simulink model "B2B_spv"  (R2017a)
settings: Solver=VariableStepAuto  StartTime=0.0  StopTime=.2  MaxStep=1e-4  RelTol=1e-3
libraries: powerlib x77, powerlib_meascontrol x11, dsparch4 x2
(part 1 of 2)
settings Model: Creator=erich  LastModifiedBy=erich

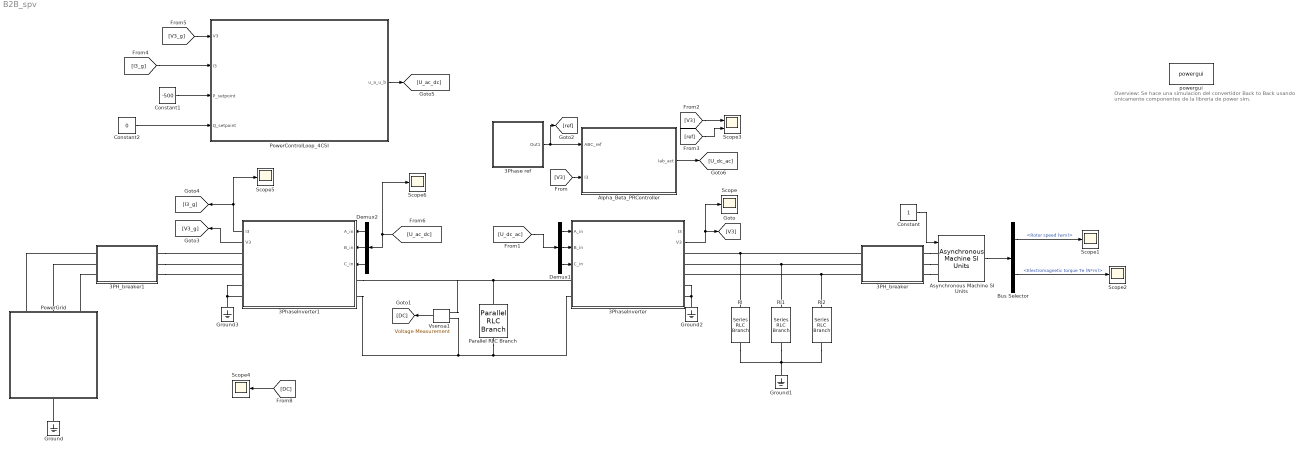
== system B2B_spv ==
  note: Overview:
      | Se hace una simulacion del convertidor
      | Back to Back usando unicamente componentes de la
      | libreria de power sim.
  3PH_breaker : Subsystem  mask{start_time=.3}
      mask prompts: start_time "Time Before  Conection"
      mask Display:
      | port_label('lconn', 1, 'a')
      | port_label('lconn', 2, 'b')
      | port_label('lconn', 3, 'c')
      | port_label('rconn', 1, 'A')
      | port_label('rconn', 2, 'B')
      | port_label('rconn', 3, 'C')
      | 
      | text(.3, .3, '3 \Phi Breaker', 'texmode', 'on')
      | 
      | plot([.3 .43], [.55 .55])
      | plot([.57 .7], [.55 .55])
      | 
      | x = -.09:.01:.09;
      | y = sqrt(.1.^2 - x.^2)*1.7;
      | 
      | plot(x+.5, .55+y)
  3PH_breaker1 : Subsystem  mask{start_time=2e-3}
      mask prompts: start_time "Time Before  Conection"
      mask Display:
      | port_label('lconn', 1, 'a')
      | port_label('lconn', 2, 'b')
      | port_label('lconn', 3, 'c')
      | port_label('rconn', 1, 'A')
      | port_label('rconn', 2, 'B')
      | port_label('rconn', 3, 'C')
      | 
      | text(.3, .3, '3 \Phi Breaker', 'texmode', 'on')
      | 
      | plot([.3 .43], [.55 .55])
      | plot([.57 .7], [.55 .55])
      | 
      | x = -.09:.01:.09;
      | y = sqrt(.1.^2 - x.^2)*1.7;
      | 
      | plot(x+.5, .55+y)
  3Phase ref : Subsystem  mask{f=60, A=170}
      mask prompts: f "Frequency (Hz)"; A "Amplitude"
      mask Display:
      | port_label('output', 1, 'sine(t)_{abc}', 'texmode', 'on')
      | 
      | 
      | plot([0:.001:.3], sin([0:.001:.3]*2*pi*10)/10+.8)
      | plot([0:.001:.3], sin([0:.001:.3]*2*pi*10)/10+.5)
      | plot([0:.001:.3], sin([0:.001:.3]*2*pi*10)/10+.2)
  3PhaseInverter : Subsystem  mask(Power SIM Block){f_sw=10000, start_Delay=.3, filter=[2e-3 .01 4.7e-6 .01]}
      mask prompts: f_sw "Switching Frequency (Hz)"; start_Delay "Converter starting delay"; filter "Parametros filtros [Lf, rLf, Cf, rCf]"
      mask help: Este es un convertidor trifasico implementado a la partir de la topologia 3 leg converter. Se emplea un filtro LC trifasico para suavizar la salida del inversor. puede hacer operacion bidireccional (DC -> AC y AC -> DC).
      mask DialogControl DescTextVar Prompt: Configuracion Del Inversor Trifasico. Switching Frequency corresponde a la frecuencia de conmutacion de los transistores. El time delay corresponde a un tiempo muerto durante el inicio del convertidor en el cual todos los interruptores (que hacen las veces de IGBTs) del convertidor tendran 0 en gate, es decir el convertidor no reaccionara.
      mask Display:
      | port_label('input', 1, 'A_u', 'texmode', 'on')
      | port_label('input', 2, 'B_u', 'texmode', 'on')
      | port_label('input', 3, 'C_u', 'texmode', 'on')
      | 
      | port_label('lconn', 1, 'DC +')
      | port_label('lconn', 2, 'DC -')
      | 
      | 
      | port_label('rconn', 1, 'A')
      | port_label('rconn', 2, 'B')
      | port_label('rconn', 3, 'C')
      | port_label('rconn', 4, 'Neutral')
      | port_label('rconn', 5, 'Cap Commons')
      | 
      | port_label('output', 1, 'I_{3\Phi}', 'texmode', 'on')
      | port_label('output', 2, 'V_{3\Phi}', 'texmode', 'on')
      | 
      | plot([0.1 .9], [0.1 .9])
      | plot([0.2 .4], [.7 .7])
      | plot([0.2 .24], [.65 .65])
      | plot([0.28 .32], [.65 .65])
      | plot([0.36 .40], [.65 .65])
      | 
      | plot([.5:.01:.7], .25+sin(30*[.2:.01:.4])/10)
  3PhaseInverter1 : Subsystem  mask(Power SIM Block){f_sw=10000, start_Delay=2e-3, filter=[12e-3 1e-3 22e-6 1e-3]}
      mask prompts: f_sw "Switching Frequency (Hz)"; start_Delay "Converter starting delay"; filter "Parametros filtros [Lf, rLf, Cf, rCf]"
      mask help: Este es un convertidor trifasico implementado a la partir de la topologia 3 leg converter. Se emplea un filtro LC trifasico para suavizar la salida del inversor. puede hacer operacion bidireccional (DC -> AC y AC -> DC).
      mask DialogControl DescTextVar Prompt: Configuracion Del Inversor Trifasico. Switching Frequency corresponde a la frecuencia de conmutacion de los transistores. El time delay corresponde a un tiempo muerto durante el inicio del convertidor en el cual todos los interruptores (que hacen las veces de IGBTs) del convertidor tendran 0 en gate, es decir el convertidor no reaccionara.
      mask Display:
      | port_label('input', 1, 'A_u', 'texmode', 'on')
      | port_label('input', 2, 'B_u', 'texmode', 'on')
      | port_label('input', 3, 'C_u', 'texmode', 'on')
      | 
      | port_label('lconn', 1, 'DC +')
      | port_label('lconn', 2, 'DC -')
      | 
      | 
      | port_label('rconn', 1, 'A')
      | port_label('rconn', 2, 'B')
      | port_label('rconn', 3, 'C')
      | port_label('rconn', 4, 'Neutral')
      | port_label('rconn', 5, 'Cap Commons')
      | 
      | port_label('output', 1, 'I_{3\Phi}', 'texmode', 'on')
      | port_label('output', 2, 'V_{3\Phi}', 'texmode', 'on')
      | 
      | plot([0.1 .9], [0.1 .9])
      | plot([0.2 .4], [.7 .7])
      | plot([0.2 .24], [.65 .65])
      | plot([0.28 .32], [.65 .65])
      | plot([0.36 .40], [.65 .65])
      | 
      | plot([.5:.01:.7], .25+sin(30*[.2:.01:.4])/10)
  Alpha_Beta_PRController : Subsystem  mask{Kp=.0002/100, Ki=.5, w0=2*pi*60, wa=.1, start_delay=2e-3}
      mask prompts: Kp "Ganancia Proporcional"; Ki "Ganancia Integral"; w0 "Frencuencia Central"; wa "Ancho de campana de resonancia"; start_delay "Retardo Calculo Accion de Control"
      mask Display:
      | port_label('input', 1, '\fontsize{13} [A, B, C]_{ref}', 'texmode', 'on')
      | %port_label('input', 2, '\fontsize{13} \beta_{ref}', 'texmode', 'on')
      | port_label('input', 2, '\fontsize{13} [ A, B, C ]_{meas}', 'texmode', 'on')
      | 
      | port_label('output', 1, '\fontsize{13} [ u_{a}, u_{b}, u_{c} ]', 'texmode', 'on')
      | 
      | 
      | %plot([.4 .6],.05+[.5 .7])
      | %plot([.4 .6],.05+[.9 .7])
      | %plot([.4 .4],.05+[.9 .5])
      | 
      | text(.53,.2,'\fontsize{25} \int', 'texmode', 'on')
      | plot(.65+[0:.01:pi/10], .2+sin(40*[0:.01:pi/10])/13)
      | 
      | %text(.5,.8,'\fontsize{15} PR_{\alpha \beta}', 'texmode', 'on')
  Asynchronous Machine SI Units : powerlib/Machines/Asynchronous Machine SI Units  RotorType=Squirrel-cage  PresetModel=No  MechanicalLoad=Torque Tm  ShowDetailedParameters=on  ReferenceFrame=Rotor  Units=SI  MeasurementBus=off  NominalParameters=[1.845e+04 200 60]  Stator=[0.5968 0.0003495]  Rotor=[0.6258 0.005473]  Cage1=[0.4155 0.002066]  Cage2=[0.4168 0.0003495]  Lm=0.0354  Mechanical=[0.00007 0.00879 2]  PolePairs=2  InitialConditions=[0 0 0 0 0 0 0 0]  SimulateSaturation=off  Saturation=[14.03593122, 27.81365428, 53.79336849, 72.68890987, 97.98006896, 148.6815601, 215.7428561, 302.9841135, 428.7778367 ; 230, 322, 414, 460, 506, 552, 598, 644, 690]  LoadFlowParameters=1492000  TsPowergui=0  TsBlock=-1  IterativeModel=Trapezoidal non iterative  IterativeDiscreteModel=Trapezoidal non iterative  Pmec=1.492e+006
  Bus Selector : BusSelector  OutputSignals=Mechanical.Rotor speed (wm),Mechanical.Electromagnetic torque Te (N*m)
  Constant : Constant
  Constant1 : Constant  Value=-500
  Constant2 : Constant  Value=0
  Demux1 : Demux  Outputs=3
  Demux2 : Demux  Outputs=3
  Ground{,1..3} (4 alike) : powerlib/Elements/Ground  LConnTagsString=a
  Parallel RLC Branch : powerlib/Elements/Parallel RLC Branch  LConnTagsString=a  RConnTagsString=__new0  BranchType=RC  Resistance=1e6  Inductance=1e-3  SetiL0=off  InitialCurrent=0  Capacitance=10000e-6  Setx0=on  InitialVoltage=0  Measurements=None
  PowerControlLoop_4CSI : Subsystem  mask{Kp=2/100, Ki=2, wa=100, w0=2*pi*60, start_delay=2e-3}
      mask prompts: Kp "Kp Controller Proportinal gain"; Ki "Ki Controller integral gain"; wa "Ancho campana"; w0 "Frecuencia central (rads/seg)"; start_delay "Start Delay"
      mask Display:
      | port_label('input', 1, '\fontsize{14} V_{abc}', 'texmode', 'on')
      | port_label('input', 2, '\fontsize{14} I_{abc}', 'texmode', 'on')
      | port_label('input', 3, '\fontsize{14} P_{set}', 'texmode', 'on')
      | port_label('input', 4, '\fontsize{14} Q_{set}', 'texmode', 'on')
      | port_label('output', 1, '\fontsize{14} u_{a, b, c}', 'texmode', 'on')
      | 
      | 
      | disp('\fontsize{12} Power Control for 3\Phi CSI', 'texmode', 'on')
  PowerGrid : Subsystem  mask{A=170, f=60, r=0, L=1e-9}
      mask prompts: A "Amplitude Voltage (Volts)"; f "Frequency (Hz)"; r "Resistance series impedance"; L "Inductance series impedance"
      mask Display:
      | port_label('lconn', 1, 'A')
      | port_label('lconn', 2, 'B')
      | port_label('lconn', 3, 'C')
      | 
      | port_label('rconn', 1, 'GND')
      | 
      | 
      | plot([.32 .4],[.2 .3])
      | plot([.32 .5],[.2 .3])
      | 
      | plot([.68 .6],[.2 .3])
      | plot([.68 .5],[.2 .3])
      | 
      | plot([.4 .6], [.3 .3])
      | plot([.4 .4], [.3 .42])
      | plot([.6 .6], [.3 .42])
      | plot([.4 .6], [.42 .42])
      | 
      | plot([.4 .6], [.3 .42])
      | plot([.6 .4], [.3 .42])
      | 
      | plot([.4 .44], [.42 .65])
      | plot([.6 .56], [.42 .65])
      | 
      | plot([.4 .56], [.42 .65])
      | plot([.6 .44], [.42 .65])
      | 
      | plot([.44 .56], [.65 .65])
      | 
      | plot([.44 .44], [.65 .78])
      | plot([.56 .56], [.65 .78])
      | 
      | plot([.44 .56], [.78 .78])
      | 
      | plot([.44 .5], [.78 .85])
      | plot([.56 .5], [.78 .85])
      | 
      | plot([.2 .8], [.69 .69])
      | plot([.2 .8], [.725 .725])
      | plot([.2 .8], [.76 .76])
      | 
      | % raulest50@gmail.com
  Rl : powerlib/Elements/Series RLC Branch  LConnTagsString=__new0  RConnTagsString=__new0  BranchType=R  Resistance=150  Inductance=1e-3  SetiL0=off  InitialCurrent=0  Capacitance=1e-6  Setx0=off  InitialVoltage=0  Measurements=None
  Rl1 : powerlib/Elements/Series RLC Branch  LConnTagsString=__new0  RConnTagsString=__new0  BranchType=R  Resistance=150  Inductance=1e-3  SetiL0=off  InitialCurrent=0  Capacitance=1e-6  Setx0=off  InitialVoltage=0  Measurements=None
  Rl2 : powerlib/Elements/Series RLC Branch  LConnTagsString=__new0  RConnTagsString=__new0  BranchType=R  Resistance=150  Inductance=1e-3  SetiL0=off  InitialCurrent=0  Capacitance=1e-6  Setx0=off  InitialVoltage=0  Measurements=None
  Scope{,1..2,4..6} (6 alike) : Scope
  Scope3 : Scope  NumInputPorts=2
  Vsensa1 : powerlib/Measurements/Voltage Measurement  PhasorSimulation=off  OutputType=Complex  PSBequivalent=0
  powergui : powerlib/powergui  Priority=1  SimulationMode=Continuous  SampleTime=50e-6  frequency=60  Iterations=50  frequencyindice=0  Pbase=100e6  ErrMax=1e-4  UnitsV=kV  UnitsW=MW  buscounter=0  FunctionMessages=off  echomessages=off  EnableUseOfTLC=off  CurrentSourceSwitches=off  DisableSnubberDevices=off  DisableRonSwitches=off  DisableVfSwitches=off  DisplayEquations=off  SolverType=Tustin/Backward Euler (TBE)  Interpol=off  ExternalGateDelay=off  methode=off  Ts=100  x0status=blocks  SPID=on  SwTol=0  HookPort=off  RestoreLinks=warning  ResistiveCurrentMeasurement=off  Frange=[0:2:500]  Ylog=off  Xlog=on  ShowGrid=off  save=off  variable=ZData  structure=0  ZoomFFT=off  StartTime=0.0  cycles=1  DisplayStyle=1  fundamental=60  FreqAxis=off  MaxFrequency=1000  frequencyindicesteady=1  RmsSteady=1  display=off
  wires:
  Constant/1 -> Asynchronous Machine SI Units/1
  Asynchronous Machine SI Units/1 -> Bus Selector/1
  Bus Selector/1 -> Scope1/1  "<Rotor speed (wm)>"
  Bus Selector/2 -> Scope2/1  "<Electromagnetic torque Te (N*m)>"
  [V3] -> Alpha_Beta_PRController/2(I3)
  Alpha_Beta_PRController/1(Iab_act) -> [U_dc_ac]
  Demux1/2 -> 3PhaseInverter/2(B_in)
  Demux1/1 -> 3PhaseInverter/1(A_in)
  Demux1/3 -> 3PhaseInverter/3(C_in)
  3PhaseInverter/2(V3) -> Scope/1, [V3]
  [U_dc_ac] -> Demux1/1
  3Phase ref/1(Out1) -> [ref], Alpha_Beta_PRController/1(ABC_ref)
  [V3] -> Scope3/1
  [ref] -> Scope3/2
  3PhaseInverter1/2(V3) -> [V3_g]
  3PhaseInverter1/1(I3) -> Scope5/1, [I3_g]
  Demux2/3 -> 3PhaseInverter1/3(C_in)
  Demux2/2 -> 3PhaseInverter1/2(B_in)
  Demux2/1 -> 3PhaseInverter1/1(A_in)
  [U_ac_dc] -> Scope6/1, Demux2/1
  PowerControlLoop_4CSI/1(u_a_u_b) -> [U_ac_dc]
  [V3_g] -> PowerControlLoop_4CSI/1(V3)
  [I3_g] -> PowerControlLoop_4CSI/2(I3)
  Constant1/1 -> PowerControlLoop_4CSI/3(P_setpoint)
  Constant2/1 -> PowerControlLoop_4CSI/4(Q_setpoint)
  Vsensa1/1 -> [DC]
  [DC] -> Scope4/1
  connections:
  Ground/LConn1 -- PowerGrid/RConn1
  3PhaseInverter1/LConn2 -- Vsensa1/LConn2 -- Parallel RLC Branch/LConn1 -- 3PhaseInverter/LConn2
  Parallel RLC Branch/RConn1 -- 3PhaseInverter/LConn1 -- 3PhaseInverter1/LConn1 -- Vsensa1/LConn1
  3PhaseInverter/RConn4 -- 3PhaseInverter/RConn5 -- Ground2/LConn1
  Ground1/LConn1 -- Rl2/RConn1 -- Rl1/RConn1 -- Rl/RConn1
  3PH_breaker/RConn2 -- Asynchronous Machine SI Units/LConn2
  3PH_breaker/RConn1 -- Asynchronous Machine SI Units/LConn1
  3PH_breaker/RConn3 -- Asynchronous Machine SI Units/LConn3
  3PH_breaker/LConn1 -- Rl/LConn1 -- 3PhaseInverter/RConn1
  3PH_breaker/LConn2 -- Rl1/LConn1 -- 3PhaseInverter/RConn2
  3PH_breaker/LConn3 -- Rl2/LConn1 -- 3PhaseInverter/RConn3
  3PhaseInverter1/RConn4 -- 3PhaseInverter1/RConn5 -- Ground3/LConn1
  3PH_breaker1/LConn3 -- PowerGrid/LConn3
  3PH_breaker1/LConn2 -- PowerGrid/LConn2
  3PH_breaker1/LConn1 -- PowerGrid/LConn1
  3PH_breaker1/RConn1 -- 3PhaseInverter1/RConn1
  3PH_breaker1/RConn2 -- 3PhaseInverter1/RConn2
  3PH_breaker1/RConn3 -- 3PhaseInverter1/RConn3

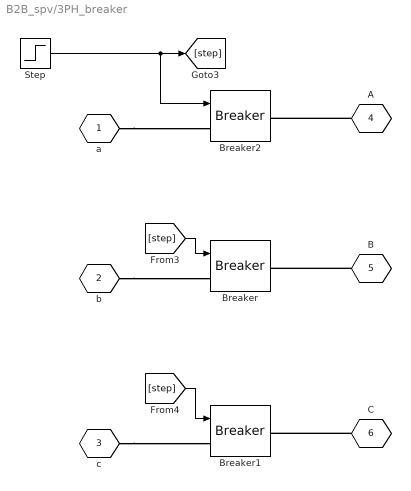
== system B2B_spv/3PH_breaker ==
  Breaker : powerlib/Elements/Breaker  InitialState=0  SwitchingTimes="[1/60  5/60]"  External=on  BreakerResistance=0.01  SnubberResistance=1e6  SnubberCapacitance=inf  Measurements=None  MoreParameters=on  NoBreakLoop=off
      settings: SourceProductName=Simscape Power Systems
  Breaker1 : powerlib/Elements/Breaker  InitialState=0  SwitchingTimes="[1/60  5/60]"  External=on  BreakerResistance=0.01  SnubberResistance=1e6  SnubberCapacitance=inf  Measurements=None  MoreParameters=on  NoBreakLoop=off
      settings: SourceProductName=Simscape Power Systems
  Breaker2 : powerlib/Elements/Breaker  InitialState=0  SwitchingTimes="[1/60  5/60]"  External=on  BreakerResistance=0.01  SnubberResistance=1e6  SnubberCapacitance=inf  Measurements=None  MoreParameters=on  NoBreakLoop=off
      settings: SourceProductName=Simscape Power Systems
  Step : Step  Time=start_time  SampleTime=0
  a : PMIOPort  Tag=PMCPort  Port=1  Side=Left
  b : PMIOPort  Tag=PMCPort  Port=2  Side=Left
  c : PMIOPort  Tag=PMCPort  Port=3  Side=Left
  A : PMIOPort  Tag=PMCPort  Port=4  Side=Right
  B : PMIOPort  Tag=PMCPort  Port=5  Side=Right
  C : PMIOPort  Tag=PMCPort  Port=6  Side=Right
  wires:
  Step/1 -> Breaker2/1, [step]
  [step] -> Breaker1/1
  [step] -> Breaker/1
  connections:
  A/RConn1 -- Breaker2/RConn1
  B/RConn1 -- Breaker/RConn1
  c/RConn1 -- Breaker1/LConn1
  C/RConn1 -- Breaker1/RConn1
  b/RConn1 -- Breaker/LConn1
  a/RConn1 -- Breaker2/LConn1

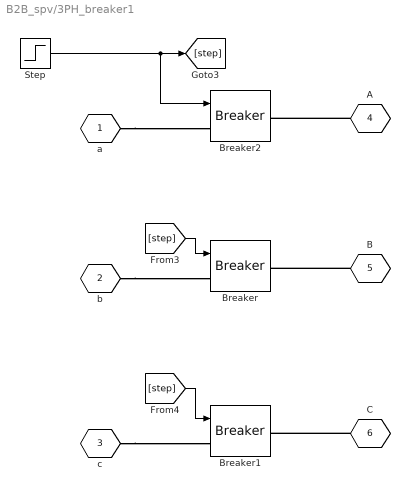
== system B2B_spv/3PH_breaker1 ==
  Breaker : powerlib/Elements/Breaker  InitialState=0  SwitchingTimes="[1/60  5/60]"  External=on  BreakerResistance=0.01  SnubberResistance=1e6  SnubberCapacitance=inf  Measurements=None  MoreParameters=on  NoBreakLoop=off
      settings: SourceProductName=Simscape Power Systems
  Breaker1 : powerlib/Elements/Breaker  InitialState=0  SwitchingTimes="[1/60  5/60]"  External=on  BreakerResistance=0.01  SnubberResistance=1e6  SnubberCapacitance=inf  Measurements=None  MoreParameters=on  NoBreakLoop=off
      settings: SourceProductName=Simscape Power Systems
  Breaker2 : powerlib/Elements/Breaker  InitialState=0  SwitchingTimes="[1/60  5/60]"  External=on  BreakerResistance=0.01  SnubberResistance=1e6  SnubberCapacitance=inf  Measurements=None  MoreParameters=on  NoBreakLoop=off
      settings: SourceProductName=Simscape Power Systems
  Step : Step  Time=start_time  SampleTime=0
  a : PMIOPort  Tag=PMCPort  Port=1  Side=Left
  b : PMIOPort  Tag=PMCPort  Port=2  Side=Left
  c : PMIOPort  Tag=PMCPort  Port=3  Side=Left
  A : PMIOPort  Tag=PMCPort  Port=4  Side=Right
  B : PMIOPort  Tag=PMCPort  Port=5  Side=Right
  C : PMIOPort  Tag=PMCPort  Port=6  Side=Right
  wires:
  Step/1 -> Breaker2/1, [step]
  [step] -> Breaker1/1
  [step] -> Breaker/1
  connections:
  A/RConn1 -- Breaker2/RConn1
  B/RConn1 -- Breaker/RConn1
  c/RConn1 -- Breaker1/LConn1
  C/RConn1 -- Breaker1/RConn1
  b/RConn1 -- Breaker/LConn1
  a/RConn1 -- Breaker2/LConn1

== system B2B_spv/3Phase ref ==
  note: Este bloque se usa para crear
      | señales de referencia arbitrarias
      | para un sistema trifasico.
  Bus Creator : BusCreator  Inputs='A','B','C'
  Sine Wave1 : Sin  Amplitude=A  Frequency=2*pi*f
  Sine Wave2 : Sin  Amplitude=A  Frequency=2*pi*f  Phase=2*pi/3
  Sine Wave3 : Sin  Amplitude=A  Frequency=2*pi*f  Phase=-2*pi/3
  Out1 : Outport
  wires:
  Sine Wave3/1 -> Bus Creator/3  "C"
  Sine Wave2/1 -> Bus Creator/2  "B"
  Bus Creator/1 -> Out1/1
  Sine Wave1/1 -> Bus Creator/1  "A"

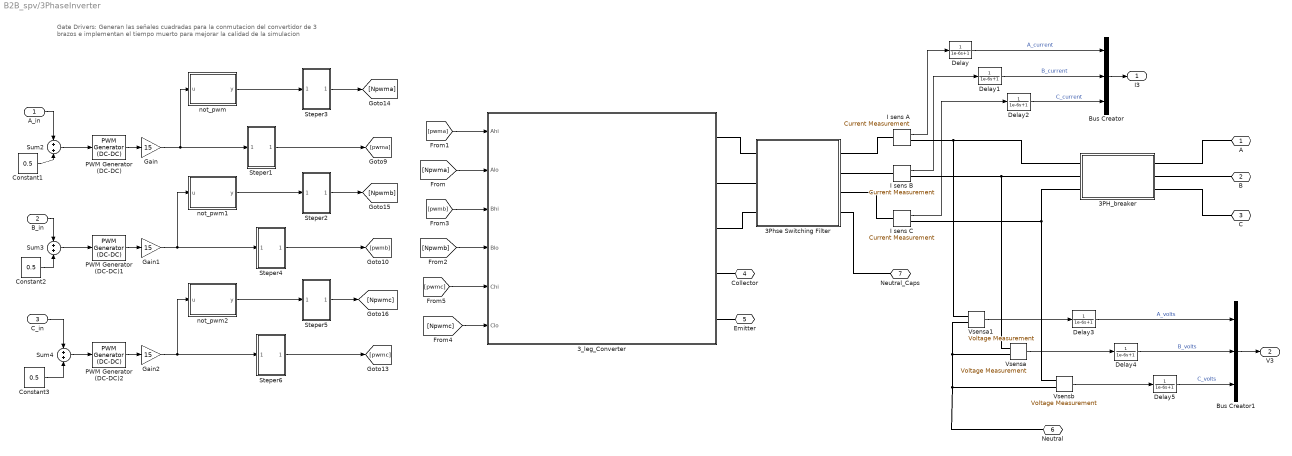
== system B2B_spv/3PhaseInverter ==
  note: Gate Drivers: Generan las señales cuadradas para
      | la conmutacion del convertidor de 3 brazos e implementan el
      | tiempo muerto para mejorar la calidad de la simulacion
  A_in : Inport
  B_in : Inport  Port=2
  C_in : Inport  Port=3
  3PH_breaker : Subsystem  mask{start_time=start_Delay}
      mask prompts: start_time "Time Before  Conection"
      mask Display:
      | port_label('lconn', 1, 'a')
      | port_label('lconn', 2, 'b')
      | port_label('lconn', 3, 'c')
      | port_label('rconn', 1, 'A')
      | port_label('rconn', 2, 'B')
      | port_label('rconn', 3, 'C')
      | 
      | text(.3, .3, '3 \Phi Breaker', 'texmode', 'on')
      | 
      | plot([.3 .43], [.55 .55])
      | plot([.57 .7], [.55 .55])
      | 
      | x = -.09:.01:.09;
      | y = sqrt(.1.^2 - x.^2)*1.7;
      | 
      | plot(x+.5, .55+y)
  3Phse Switching Filter : Subsystem  mask{Lf=filter(1), rLf=filter(2), Cf=filter(3), rCf=filter(4)}
      mask prompts: Lf "Inductancia (H)"; rLf "Resistencia parasita serie L (Ohm)"; Cf "Capacitancia (f)"; rCf "Resistencia parasita C serie"
      mask DialogControl DescTextVar Prompt: Configuracion del Filtro LC
      mask Display:
      | port_label('lconn', 1, 'A_{in}', 'texmode', 'on')
      | port_label('lconn', 2, 'B_{in}', 'texmode', 'on')
      | port_label('lconn', 3, 'B_{in}', 'texmode', 'on')
      | port_label('rconn', 1, 'A_{out}', 'texmode', 'on')
      | port_label('rconn', 2, 'B_{out}', 'texmode', 'on')
      | port_label('rconn', 3, 'C_{out}', 'texmode', 'on')
      | 
      | 
      | plot([.2 .5], [.7 .7])
      | plot([.5 .6], [.7 .3])
      | plot([.6 .7], [.3 .3])
      | 
      | text(.2, .8, '\fontsize{12} H(\omega)', 'texmode', 'on')
      | text(.6, .25, '\fontsize{12} \omega', 'texmode', 'on')
  3_leg_Converter : Subsystem
      mask Display:
      | port_label('input', 1, 'Ahi')
      | port_label('input', 2, 'Alo')
      | port_label('input', 3, 'Bhi')
      | port_label('input', 4, 'Blo')
      | port_label('input', 5, 'Chi')
      | port_label('input', 6, 'Clo')
      | 
      | port_label('rconn', 1, 'A')
      | port_label('rconn', 2, 'B')
      | port_label('rconn', 3, 'C')
      | port_label('rconn', 4, 'Collector')
      | port_label('rconn', 5, 'Emitter')
      | 
      | lvx = [.1 .1];
      | lvy = [.1 .2];
      | lhx = [.1 .2];
      | lhy = [.1 .1];
      | 
      | 
      | % se dibujan los interruptores de la izquierda
      | plot(lvx+.07, lvy*.8+.028+.1)
      | plot(lvx+.1, lvy+.1)
      | plot(lhx*.5+.15, lhy+.1)
      | plot(lhx*.5+.15, lhy+.2)
      | plot(lhx*.5+.07, lhy+.15)
      | 
      | d=0.5;
      | 
      | plot(lvx+.07, lvy*.8+.028+.1+d)
      | plot(lvx+.1, lvy+.1+d)
      | plot(lhx*.5+.15, lhy+.1+d)
      | plot(lhx*.5+.15, lhy+.2+d)
      | plot(lhx*.5+.07, lhy+.15+d)
      | 
      | 
      | % se dibujan los interruptores del medio
      | h=.3;
      | 
      | plot(lvx+.07+h, lvy*.8+.028+.1)
      | plot(lvx+.1+h, lvy+.1)
      | plot(lhx*.5+.15+h, lhy+.1)
      | plot(lhx*.5+.15+h, lhy+.2)
      | plot(lhx*.5+.07+h, lhy+.15)
      | 
      | plot(lvx+.07+h, lvy*.8+.028+.1+d)
      | plot(lvx+.1+h, lvy+.1+d)
      | plot(lhx*.5+.15+h, lhy+.1+d)
      | plot(lhx*.5+.15+h, lhy+.2+d)
      | plot(lhx*.5+.07+h, lhy+.15+d)
      | 
      | % se dibujan los interruptores de la derecha
      | h=.6
      | 
      | plot(lvx+.07+h, lvy*.8+.028+.1)
      | plot(lvx+.1+h, lvy+.1)
      | plot(lhx*.5+.15+h, lhy+.1)
      | plot(lhx*.5+.15+h, lhy+.2)
      | plot(lhx*.5+.07+h, lhy+.15)
      | 
      | plot(lvx+.07+h, lvy*.8+.028+.1+d)
      | plot(lvx+.1+h, lvy+.1+d)
      | plot(lhx*.5+.15+h, lhy+.1+d)
      | plot(lhx*.5+.15+h, lhy+.2+d)
      | plot(lhx*.5+.07+h, lhy+.15+d)
      | 
      | 
      | % se conectan los interruptores.
      | plot(lvx+.15, lvy*4-.1)
      | plot(lvx+.15+.3, lvy*4-.1)
      | plot(lvx+.15+.6, lvy*4-.1)
      | 
      | 
      | plot(lvx+.15, lvy+.7)
      | plot(lvx+.15+.3, lvy+.7)
      | plot(lvx+.15+.6, lvy+.7)
      | 
      | plot(lvx+.15, lvy)
      | plot(lvx+.15+.3, lvy)
      | plot(lvx+.15+.6, lvy)
      | 
      | plot(lhx*6-.35, lhy)
      | plot(lhx*6-.35, lhy+.8)
      | 
      | % raul esteban alzate 313 515 86 11
  Bus Creator : BusCreator  Inputs='A_current','B_current','C_current'
  Bus Creator1 : BusCreator  Inputs='A_volts','B_volts','C_volts'
  Constant1 : Constant  Value=0.5
  Constant2 : Constant  Value=0.5
  Constant3 : Constant  Value=0.5
  Delay{,1..5} (6 alike) : TransferFcn  Denominator=[1e-6 1]
  Gain : Gain  Gain=15
  Gain1 : Gain  Gain=15
  Gain2 : Gain  Gain=15
  I sens A : powerlib/Measurements/Current Measurement  PhasorSimulation=off  OutputType=Complex  PSBequivalent=0
  I sens B : powerlib/Measurements/Current Measurement  PhasorSimulation=off  OutputType=Complex  PSBequivalent=0
  I sens C : powerlib/Measurements/Current Measurement  PhasorSimulation=off  OutputType=Complex  PSBequivalent=0
  PWM Generator (DC-DC) : powerlib_meascontrol/Pulse & Signal Generators/PWM Generator (DC-DC)  Fsw=f_sw  Ts=0
  PWM Generator (DC-DC)1 : powerlib_meascontrol/Pulse & Signal Generators/PWM Generator (DC-DC)  Fsw=f_sw  Ts=0
  PWM Generator (DC-DC)2 : powerlib_meascontrol/Pulse & Signal Generators/PWM Generator (DC-DC)  Fsw=f_sw  Ts=0
  Steper1 : Subsystem
  Steper2 : Subsystem
  Steper3 : Subsystem
  Steper4 : Subsystem
  Steper5 : Subsystem
  Steper6 : Subsystem
  Sum2 : Sum
  Sum3 : Sum
  Sum4 : Sum
  Vsensa : powerlib/Measurements/Voltage Measurement  PhasorSimulation=off  OutputType=Complex  PSBequivalent=0
  Vsensa1 : powerlib/Measurements/Voltage Measurement  PhasorSimulation=off  OutputType=Complex  PSBequivalent=0
  Vsensb : powerlib/Measurements/Voltage Measurement  PhasorSimulation=off  OutputType=Complex  PSBequivalent=0
  not_pwm : MATLAB Function  TreatAsAtomicUnit=on
  not_pwm1 : MATLAB Function  TreatAsAtomicUnit=on
  not_pwm2 : MATLAB Function  TreatAsAtomicUnit=on
  A : PMIOPort  Port=1  Side=Right
  B : PMIOPort  Port=2  Side=Right
  C : PMIOPort  Port=3  Side=Right
  Collector : PMIOPort  Port=4  Side=Left
  Emitter : PMIOPort  Port=5  Side=Left
  Neutral : PMIOPort  Port=6  Side=Right
  Neutral_Caps : PMIOPort  Port=7  Side=Right
  I3 : Outport
  V3 : Outport  Port=2
  wires:
  Steper4/1(Out1) -> [pwmb]
  Gain1/1 -> Steper4/1(In1), not_pwm1/1(u)
  not_pwm1/1(y) -> Steper2/1(In1)
  PWM Generator (DC-DC)2/1 -> Gain2/1
  Sum4/1 -> PWM Generator (DC-DC)2/1
  not_pwm/1(y) -> Steper3/1(In1)
  Constant3/1 -> Sum4/2
  PWM Generator (DC-DC)1/1 -> Gain1/1
  not_pwm2/1(y) -> Steper5/1(In1)
  C_in/1 -> Sum4/1
  Sum2/1 -> PWM Generator (DC-DC)/1
  I sens C/1 -> Delay2/1
  PWM Generator (DC-DC)/1 -> Gain/1
  B_in/1 -> Sum3/1
  Constant1/1 -> Sum2/2
  Steper2/1(Out1) -> [Npwmb]
  A_in/1 -> Sum2/1
  I sens A/1 -> Delay/1
  Bus Creator/1 -> I3/1
  Sum3/1 -> PWM Generator (DC-DC)1/1
  Gain2/1 -> Steper6/1(In1), not_pwm2/1(u)
  Steper5/1(Out1) -> [Npwmc]
  Steper1/1(Out1) -> [pwma]
  I sens B/1 -> Delay1/1
  Constant2/1 -> Sum3/2
  Steper3/1(Out1) -> [Npwma]
  Gain/1 -> Steper1/1(In1), not_pwm/1(u)
  Steper6/1(Out1) -> [pwmc]
  Vsensb/1 -> Delay5/1
  Bus Creator1/1 -> V3/1
  Vsensa/1 -> Delay4/1
  Vsensa1/1 -> Delay3/1
  [pwma] -> 3_leg_Converter/1(Ahi)
  [Npwma] -> 3_leg_Converter/2(Alo)
  [pwmb] -> 3_leg_Converter/3(Bhi)
  [Npwmb] -> 3_leg_Converter/4(Blo)
  [pwmc] -> 3_leg_Converter/5(Chi)
  [Npwmc] -> 3_leg_Converter/6(Clo)
  Delay/1 -> Bus Creator/1  "A_current"
  Delay1/1 -> Bus Creator/2  "B_current"
  Delay2/1 -> Bus Creator/3  "C_current"
  Delay3/1 -> Bus Creator1/1  "A_volts"
  Delay4/1 -> Bus Creator1/2  "B_volts"
  Delay5/1 -> Bus Creator1/3  "C_volts"
  connections:
  3Phse Switching Filter/LConn2 -- 3_leg_Converter/RConn2
  I sens B/LConn1 -- 3Phse Switching Filter/RConn2
  Vsensa1/LConn1 -- 3PH_breaker/LConn1 -- I sens A/RConn1
  3Phse Switching Filter/LConn3 -- 3_leg_Converter/RConn3
  I sens A/LConn1 -- 3Phse Switching Filter/RConn1
  Vsensa/LConn1 -- I sens B/RConn1 -- 3PH_breaker/LConn2
  3Phse Switching Filter/LConn1 -- 3_leg_Converter/RConn1
  Vsensb/LConn1 -- 3PH_breaker/LConn3 -- I sens C/RConn1
  I sens C/LConn1 -- 3Phse Switching Filter/RConn3
  Vsensa/LConn2 -- Vsensa1/LConn2 -- Neutral/RConn1 -- Vsensb/LConn2
  3_leg_Converter/RConn4 -- Collector/RConn1
  3_leg_Converter/RConn5 -- Emitter/RConn1
  3Phse Switching Filter/RConn4 -- Neutral_Caps/RConn1
  3PH_breaker/RConn2 -- B/RConn1
  3PH_breaker/RConn1 -- A/RConn1
  C/RConn1 -- 3PH_breaker/RConn3

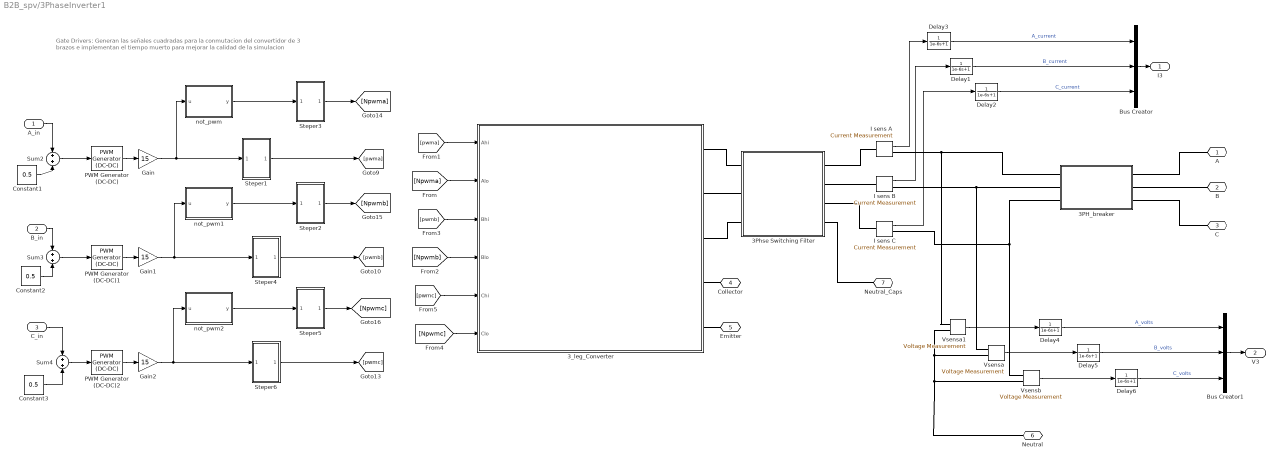
== system B2B_spv/3PhaseInverter1 ==
  note: Gate Drivers: Generan las señales cuadradas para
      | la conmutacion del convertidor de 3 brazos e implementan el
      | tiempo muerto para mejorar la calidad de la simulacion
  A_in : Inport
  B_in : Inport  Port=2
  C_in : Inport  Port=3
  3PH_breaker : Subsystem  mask{start_time=start_Delay}
      mask prompts: start_time "Time Before  Conection"
      mask Display:
      | port_label('lconn', 1, 'a')
      | port_label('lconn', 2, 'b')
      | port_label('lconn', 3, 'c')
      | port_label('rconn', 1, 'A')
      | port_label('rconn', 2, 'B')
      | port_label('rconn', 3, 'C')
      | 
      | text(.3, .3, '3 \Phi Breaker', 'texmode', 'on')
      | 
      | plot([.3 .43], [.55 .55])
      | plot([.57 .7], [.55 .55])
      | 
      | x = -.09:.01:.09;
      | y = sqrt(.1.^2 - x.^2)*1.7;
      | 
      | plot(x+.5, .55+y)
  3Phse Switching Filter : Subsystem  mask{Lf=filter(1), rLf=filter(2), Cf=filter(3), rCf=filter(4)}
      mask prompts: Lf "Inductancia (H)"; rLf "Resistencia parasita serie L (Ohm)"; Cf "Capacitancia (f)"; rCf "Resistencia parasita C serie"
      mask DialogControl DescTextVar Prompt: Configuracion del Filtro LC
      mask Display:
      | port_label('lconn', 1, 'A_{in}', 'texmode', 'on')
      | port_label('lconn', 2, 'B_{in}', 'texmode', 'on')
      | port_label('lconn', 3, 'B_{in}', 'texmode', 'on')
      | port_label('rconn', 1, 'A_{out}', 'texmode', 'on')
      | port_label('rconn', 2, 'B_{out}', 'texmode', 'on')
      | port_label('rconn', 3, 'C_{out}', 'texmode', 'on')
      | 
      | 
      | plot([.2 .5], [.7 .7])
      | plot([.5 .6], [.7 .3])
      | plot([.6 .7], [.3 .3])
      | 
      | text(.2, .8, '\fontsize{12} H(\omega)', 'texmode', 'on')
      | text(.6, .25, '\fontsize{12} \omega', 'texmode', 'on')
  3_leg_Converter : Subsystem
      mask Display:
      | port_label('input', 1, 'Ahi')
      | port_label('input', 2, 'Alo')
      | port_label('input', 3, 'Bhi')
      | port_label('input', 4, 'Blo')
      | port_label('input', 5, 'Chi')
      | port_label('input', 6, 'Clo')
      | 
      | port_label('rconn', 1, 'A')
      | port_label('rconn', 2, 'B')
      | port_label('rconn', 3, 'C')
      | port_label('rconn', 4, 'Collector')
      | port_label('rconn', 5, 'Emitter')
      | 
      | lvx = [.1 .1];
      | lvy = [.1 .2];
      | lhx = [.1 .2];
      | lhy = [.1 .1];
      | 
      | 
      | % se dibujan los interruptores de la izquierda
      | plot(lvx+.07, lvy*.8+.028+.1)
      | plot(lvx+.1, lvy+.1)
      | plot(lhx*.5+.15, lhy+.1)
      | plot(lhx*.5+.15, lhy+.2)
      | plot(lhx*.5+.07, lhy+.15)
      | 
      | d=0.5;
      | 
      | plot(lvx+.07, lvy*.8+.028+.1+d)
      | plot(lvx+.1, lvy+.1+d)
      | plot(lhx*.5+.15, lhy+.1+d)
      | plot(lhx*.5+.15, lhy+.2+d)
      | plot(lhx*.5+.07, lhy+.15+d)
      | 
      | 
      | % se dibujan los interruptores del medio
      | h=.3;
      | 
      | plot(lvx+.07+h, lvy*.8+.028+.1)
      | plot(lvx+.1+h, lvy+.1)
      | plot(lhx*.5+.15+h, lhy+.1)
      | plot(lhx*.5+.15+h, lhy+.2)
      | plot(lhx*.5+.07+h, lhy+.15)
      | 
      | plot(lvx+.07+h, lvy*.8+.028+.1+d)
      | plot(lvx+.1+h, lvy+.1+d)
      | plot(lhx*.5+.15+h, lhy+.1+d)
      | plot(lhx*.5+.15+h, lhy+.2+d)
      | plot(lhx*.5+.07+h, lhy+.15+d)
      | 
      | % se dibujan los interruptores de la derecha
      | h=.6
      | 
      | plot(lvx+.07+h, lvy*.8+.028+.1)
      | plot(lvx+.1+h, lvy+.1)
      | plot(lhx*.5+.15+h, lhy+.1)
      | plot(lhx*.5+.15+h, lhy+.2)
      | plot(lhx*.5+.07+h, lhy+.15)
      | 
      | plot(lvx+.07+h, lvy*.8+.028+.1+d)
      | plot(lvx+.1+h, lvy+.1+d)
      | plot(lhx*.5+.15+h, lhy+.1+d)
      | plot(lhx*.5+.15+h, lhy+.2+d)
      | plot(lhx*.5+.07+h, lhy+.15+d)
      | 
      | 
      | % se conectan los interruptores.
      | plot(lvx+.15, lvy*4-.1)
      | plot(lvx+.15+.3, lvy*4-.1)
      | plot(lvx+.15+.6, lvy*4-.1)
      | 
      | 
      | plot(lvx+.15, lvy+.7)
      | plot(lvx+.15+.3, lvy+.7)
      | plot(lvx+.15+.6, lvy+.7)
      | 
      | plot(lvx+.15, lvy)
      | plot(lvx+.15+.3, lvy)
      | plot(lvx+.15+.6, lvy)
      | 
      | plot(lhx*6-.35, lhy)
      | plot(lhx*6-.35, lhy+.8)
      | 
      | % raul esteban alzate 313 515 86 11
  Bus Creator : BusCreator  Inputs='A_current','B_current','C_current'
  Bus Creator1 : BusCreator  Inputs='A_volts','B_volts','C_volts'
  Constant1 : Constant  Value=0.5
  Constant2 : Constant  Value=0.5
  Constant3 : Constant  Value=0.5
  Delay{1..6} (6 alike) : TransferFcn  Denominator=[1e-6 1]
  Gain : Gain  Gain=15
  Gain1 : Gain  Gain=15
  Gain2 : Gain  Gain=15
  I sens A : powerlib/Measurements/Current Measurement  PhasorSimulation=off  OutputType=Complex  PSBequivalent=0
  I sens B : powerlib/Measurements/Current Measurement  PhasorSimulation=off  OutputType=Complex  PSBequivalent=0
  I sens C : powerlib/Measurements/Current Measurement  PhasorSimulation=off  OutputType=Complex  PSBequivalent=0
  PWM Generator (DC-DC) : powerlib_meascontrol/Pulse & Signal Generators/PWM Generator (DC-DC)  Fsw=f_sw  Ts=0
  PWM Generator (DC-DC)1 : powerlib_meascontrol/Pulse & Signal Generators/PWM Generator (DC-DC)  Fsw=f_sw  Ts=0
  PWM Generator (DC-DC)2 : powerlib_meascontrol/Pulse & Signal Generators/PWM Generator (DC-DC)  Fsw=f_sw  Ts=0
  Steper1 : Subsystem
  Steper2 : Subsystem
  Steper3 : Subsystem
  Steper4 : Subsystem
  Steper5 : Subsystem
  Steper6 : Subsystem
  Sum2 : Sum
  Sum3 : Sum
  Sum4 : Sum
  Vsensa : powerlib/Measurements/Voltage Measurement  PhasorSimulation=off  OutputType=Complex  PSBequivalent=0
  Vsensa1 : powerlib/Measurements/Voltage Measurement  PhasorSimulation=off  OutputType=Complex  PSBequivalent=0
  Vsensb : powerlib/Measurements/Voltage Measurement  PhasorSimulation=off  OutputType=Complex  PSBequivalent=0
  not_pwm : MATLAB Function  TreatAsAtomicUnit=on
  not_pwm1 : MATLAB Function  TreatAsAtomicUnit=on
  not_pwm2 : MATLAB Function  TreatAsAtomicUnit=on
  A : PMIOPort  Port=1  Side=Right
  B : PMIOPort  Port=2  Side=Right
  C : PMIOPort  Port=3  Side=Right
  Collector : PMIOPort  Port=4  Side=Left
  Emitter : PMIOPort  Port=5  Side=Left
  Neutral : PMIOPort  Port=6  Side=Right
  Neutral_Caps : PMIOPort  Port=7  Side=Right
  I3 : Outport
  V3 : Outport  Port=2
  wires:
  [Npwmc] -> 3_leg_Converter/6(Clo)
  [pwmc] -> 3_leg_Converter/5(Chi)
  [Npwmb] -> 3_leg_Converter/4(Blo)
  [pwmb] -> 3_leg_Converter/3(Bhi)
  [Npwma] -> 3_leg_Converter/2(Alo)
  [pwma] -> 3_leg_Converter/1(Ahi)
  Vsensa1/1 -> Delay4/1
  Vsensa/1 -> Delay5/1
  Bus Creator1/1 -> V3/1
  Vsensb/1 -> Delay6/1
  Steper6/1(Out1) -> [pwmc]
  Gain/1 -> not_pwm/1(u), Steper1/1(In1)
  Steper3/1(Out1) -> [Npwma]
  Constant2/1 -> Sum3/2
  I sens B/1 -> Delay1/1
  Steper1/1(Out1) -> [pwma]
  Steper5/1(Out1) -> [Npwmc]
  Gain2/1 -> not_pwm2/1(u), Steper6/1(In1)
  Sum3/1 -> PWM Generator (DC-DC)1/1
  Bus Creator/1 -> I3/1
  I sens A/1 -> Delay3/1
  A_in/1 -> Sum2/1
  Steper2/1(Out1) -> [Npwmb]
  Constant1/1 -> Sum2/2
  B_in/1 -> Sum3/1
  PWM Generator (DC-DC)/1 -> Gain/1
  I sens C/1 -> Delay2/1
  Sum2/1 -> PWM Generator (DC-DC)/1
  C_in/1 -> Sum4/1
  not_pwm2/1(y) -> Steper5/1(In1)
  PWM Generator (DC-DC)1/1 -> Gain1/1
  Constant3/1 -> Sum4/2
  not_pwm/1(y) -> Steper3/1(In1)
  Sum4/1 -> PWM Generator (DC-DC)2/1
  PWM Generator (DC-DC)2/1 -> Gain2/1
  not_pwm1/1(y) -> Steper2/1(In1)
  Gain1/1 -> not_pwm1/1(u), Steper4/1(In1)
  Steper4/1(Out1) -> [pwmb]
  Delay3/1 -> Bus Creator/1  "A_current"
  Delay1/1 -> Bus Creator/2  "B_current"
  Delay2/1 -> Bus Creator/3  "C_current"
  Delay4/1 -> Bus Creator1/1  "A_volts"
  Delay5/1 -> Bus Creator1/2  "B_volts"
  Delay6/1 -> Bus Creator1/3  "C_volts"
  connections:
  C/RConn1 -- 3PH_breaker/RConn3
  3PH_breaker/RConn1 -- A/RConn1
  3PH_breaker/RConn2 -- B/RConn1
  3Phse Switching Filter/RConn4 -- Neutral_Caps/RConn1
  3_leg_Converter/RConn5 -- Emitter/RConn1
  3_leg_Converter/RConn4 -- Collector/RConn1
  Vsensb/LConn2 -- Neutral/RConn1 -- Vsensa1/LConn2 -- Vsensa/LConn2
  I sens C/LConn1 -- 3Phse Switching Filter/RConn3
  I sens C/RConn1 -- Vsensb/LConn1 -- 3PH_breaker/LConn3
  3Phse Switching Filter/LConn1 -- 3_leg_Converter/RConn1
  I sens B/RConn1 -- Vsensa/LConn1 -- 3PH_breaker/LConn2
  I sens A/LConn1 -- 3Phse Switching Filter/RConn1
  3Phse Switching Filter/LConn3 -- 3_leg_Converter/RConn3
  3PH_breaker/LConn1 -- I sens A/RConn1 -- Vsensa1/LConn1
  I sens B/LConn1 -- 3Phse Switching Filter/RConn2
  3Phse Switching Filter/LConn2 -- 3_leg_Converter/RConn2

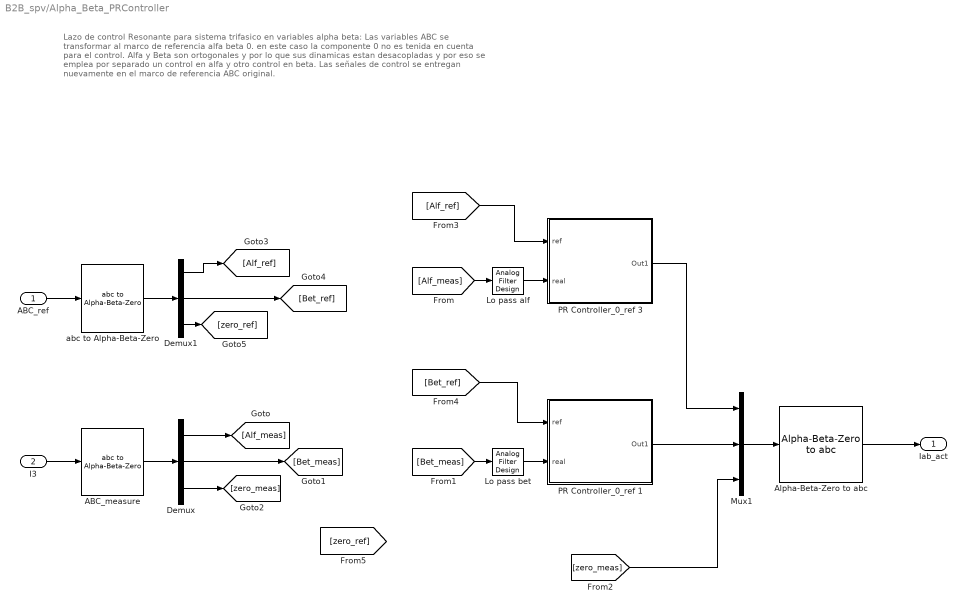
== system B2B_spv/Alpha_Beta_PRController ==
  note: Lazo de control Resonante para sistema trifasico en variables alpha beta:
      | Las variables ABC se transformar al marco de referencia alfa beta 0. en este caso la
      | componente 0 no es tenida en cuenta para el control. Alfa y Beta son ortogonales
      | y por lo que sus dinamicas estan desacopladas y por eso se emplea por separado un
      | control en alfa y otro control en beta. Las señales de control se entregan nuevamente
      | en el marco de referencia ABC original.
  ABC_ref : Inport
  I3 : Inport  Port=2
  ABC_measure : powerlib_meascontrol/Transformations/abc to Alpha-Beta-Zero
      settings: SourceProductName=Simscape Power Systems
  Alpha-Beta-Zero to abc : powerlib_meascontrol/Transformations/Alpha-Beta-Zero to abc
      settings: SourceProductName=Simscape Power Systems  SourceProductBaseCode=PS
  Demux : Demux  Outputs=3
  Demux1 : Demux  Outputs=3
  Lo pass alf : dsparch4/Analog Filter Design  method=Butterworth  filttype=Lowpass  N=1  Wlo=1000*2*pi  Whi=80  Rp=2  Rs=40
  Lo pass bet : dsparch4/Analog Filter Design  method=Butterworth  filttype=Lowpass  N=1  Wlo=1000*2*pi  Whi=80  Rp=2  Rs=40
  Mux1 : Mux  Inputs=3
  PR Controller_0_ref 1 : Subsystem  mask{Kp=Kp, Ki=Ki, wa=wa, w0=w0}
      mask prompts: Kp "Ganancia Proporcional"; Ki "Ganancia Integral"; wa "Ancho camapana resonancia"; w0 "Frecuencia Central"
      mask Display:
      | port_label('input',1,'ref')
      | port_label('input',2,'sens')
      | port_label('output',1,'out')
      | 
      | plot(.4+[0:.01:pi/10], .32+sin(40*[0:.01:pi/10])/13)
      | 
      | plot([.4 .6],.05+[.5 .7])
      | plot([.4 .6],.05+[.9 .7])
      | plot([.4 .4],.05+[.9 .5])
      | 
      | text(.27,.37,'\fontsize{25} \int', 'texmode', 'on')
  PR Controller_0_ref 3 : Subsystem  mask{Kp=Kp, Ki=Ki, wa=wa, w0=w0}
      mask prompts: Kp "Ganancia Proporcional"; Ki "Ganancia Integral"; wa "Ancho camapana resonancia"; w0 "Frecuencia Central"
      mask Display:
      | port_label('input',1,'ref')
      | port_label('input',2,'sens')
      | port_label('output',1,'out')
      | 
      | plot(.4+[0:.01:pi/10], .32+sin(40*[0:.01:pi/10])/13)
      | 
      | plot([.4 .6],.05+[.5 .7])
      | plot([.4 .6],.05+[.9 .7])
      | plot([.4 .4],.05+[.9 .5])
      | 
      | text(.27,.37,'\fontsize{25} \int', 'texmode', 'on')
  abc to Alpha-Beta-Zero : powerlib_meascontrol/Transformations/abc to Alpha-Beta-Zero
      settings: SourceProductName=Simscape Power Systems
  Iab_act : Outport
  wires:
  I3/1 -> ABC_measure/1
  PR Controller_0_ref 1/1(Out1) -> Mux1/2
  Mux1/1 -> Alpha-Beta-Zero to abc/1
  Alpha-Beta-Zero to abc/1 -> Iab_act/1
  ABC_measure/1 -> Demux/1
  PR Controller_0_ref 3/1(Out1) -> Mux1/1
  ABC_ref/1 -> abc to Alpha-Beta-Zero/1
  abc to Alpha-Beta-Zero/1 -> Demux1/1
  Demux/1 -> [Alf_meas]
  Demux/2 -> [Bet_meas]
  Demux/3 -> [zero_meas]
  [Bet_meas] -> Lo pass bet/1
  [zero_meas] -> Mux1/3
  Demux1/1 -> [Alf_ref]
  Demux1/2 -> [Bet_ref]
  Demux1/3 -> [zero_ref]
  Lo pass alf/1 -> PR Controller_0_ref 3/2(real)
  [Alf_meas] -> Lo pass alf/1
  [Alf_ref] -> PR Controller_0_ref 3/1(ref)
  Lo pass bet/1 -> PR Controller_0_ref 1/2(real)
  [Bet_ref] -> PR Controller_0_ref 1/1(ref)

== system B2B_spv/PowerControlLoop_4CSI ==
  V3 : Inport
  I3 : Inport  Port=2
  P_setpoint : Inport  Port=3
  Q_setpoint : Inport  Port=4
  Alpha_Beta_PRController : Subsystem
      mask Display:
      | port_label('input', 1, 'I_{\alpha ref}', 'texmode', 'on')
      | port_label('input', 2, 'I_{\beta ref}', 'texmode', 'on')
      | port_label('input', 3, '[ I_a, I_b, I_c ]', 'texmode', 'on')
      | 
      | port_label('output', 1, '[ I_{a act}, I_{b act}, I_{c act} ]', 'texmode', 'on')
      | 
      | plot(.65+[0:.01:pi/10], .3+sin(40*[0:.01:pi/10])/13)
      | 
      | %plot([.4 .6],.05+[.5 .7])
      | %plot([.4 .6],.05+[.9 .7])
      | %plot([.4 .4],.05+[.9 .5])
      | 
      | text(.5,.3,'\fontsize{25} \int', 'texmode', 'on')
      | 
      | text(.5,.8,'\fontsize{15} PR_{\alpha \beta}', 'texmode', 'on')
  Demux : Demux  Outputs=3
  Demux1 : Demux  Outputs=3
  Instantaneous p-q transformation : MATLAB Function  TreatAsAtomicUnit=on
  PQ2AlphBetaCurrents : MATLAB Function  TreatAsAtomicUnit=on
  u_a_u_b : Outport
  wires:
  I3/1 -> Alpha_Beta_PRController/3(I3), Demux1/1
  PQ2AlphBetaCurrents/1(Ia) -> Alpha_Beta_PRController/1(Ia_ref)
  V3/1 -> Demux/1
  Alpha_Beta_PRController/1(Iab_act) -> u_a_u_b/1
  Demux/1 -> Instantaneous p-q transformation/1(va)
  Demux1/3 -> Instantaneous p-q transformation/6(ic)
  Demux1/1 -> Instantaneous p-q transformation/4(ia)
  Demux1/2 -> Instantaneous p-q transformation/5(ib)
  P_setpoint/1 -> PQ2AlphBetaCurrents/3(p)
  Q_setpoint/1 -> PQ2AlphBetaCurrents/4(q)
  PQ2AlphBetaCurrents/2(Ib) -> Alpha_Beta_PRController/2(ib_ref)
  Demux/3 -> Instantaneous p-q transformation/3(vc)
  Instantaneous p-q transformation/9(ValA) -> PQ2AlphBetaCurrents/1(Va)
  Instantaneous p-q transformation/10(VbetA) -> PQ2AlphBetaCurrents/2(Vb)
  Demux/2 -> Instantaneous p-q transformation/2(vb)

== system B2B_spv/PowerGrid ==
  A : powerlib/Electrical Sources/AC Voltage Source  Amplitude=A  Phase=0  Frequency=f  SampleTime=0  Measurements=None  BusType=swing  Pref=10e3  Qref=0  Qmin=-inf  Qmax=+inf
  B : powerlib/Electrical Sources/AC Voltage Source  Amplitude=A  Phase=0  Frequency=f  SampleTime=0  Measurements=None  BusType=swing  Pref=10e3  Qref=0  Qmin=-inf  Qmax=+inf
  C : powerlib/Electrical Sources/AC Voltage Source  Amplitude=A  Phase=0  Frequency=f  SampleTime=0  Measurements=None  BusType=swing  Pref=10e3  Qref=0  Qmin=-inf  Qmax=+inf
  Za : powerlib/Elements/Series RLC Branch  LConnTagsString=__new0  RConnTagsString=__new0  BranchType=RL  Resistance=r  Inductance=L  SetiL0=off  InitialCurrent=0  Capacitance=0  Setx0=off  InitialVoltage=0  Measurements=None
  Zb : powerlib/Elements/Series RLC Branch  LConnTagsString=__new0  RConnTagsString=__new0  BranchType=RL  Resistance=r  Inductance=L  SetiL0=off  InitialCurrent=0  Capacitance=0  Setx0=off  InitialVoltage=0  Measurements=None
  Zc : powerlib/Elements/Series RLC Branch  LConnTagsString=__new0  RConnTagsString=__new0  BranchType=RL  Resistance=r  Inductance=L  SetiL0=off  InitialCurrent=0  Capacitance=0  Setx0=off  InitialVoltage=0  Measurements=None
  cA : PMIOPort  Port=1  Side=Left
  cB : PMIOPort  Port=2  Side=Left
  cC : PMIOPort  Port=3  Side=Left
  GND : PMIOPort  Port=4  Side=Right
  connections:
  A/LConn1 -- GND/RConn1 -- B/LConn1 -- C/LConn1
  Zb/RConn1 -- B/RConn1
  cB/RConn1 -- Zb/LConn1
  cC/RConn1 -- Zc/LConn1
  Zc/RConn1 -- C/RConn1
  Za/RConn1 -- A/RConn1
  cA/RConn1 -- Za/LConn1

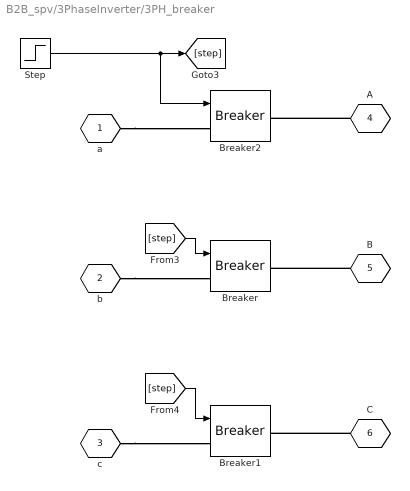
== system B2B_spv/3PhaseInverter/3PH_breaker ==
  Breaker : powerlib/Elements/Breaker  InitialState=0  SwitchingTimes="[1/60  5/60]"  External=on  BreakerResistance=0.01  SnubberResistance=1e6  SnubberCapacitance=inf  Measurements=None  MoreParameters=on  NoBreakLoop=off
      settings: SourceProductName=Simscape Power Systems
  Breaker1 : powerlib/Elements/Breaker  InitialState=0  SwitchingTimes="[1/60  5/60]"  External=on  BreakerResistance=0.01  SnubberResistance=1e6  SnubberCapacitance=inf  Measurements=None  MoreParameters=on  NoBreakLoop=off
      settings: SourceProductName=Simscape Power Systems
  Breaker2 : powerlib/Elements/Breaker  InitialState=0  SwitchingTimes="[1/60  5/60]"  External=on  BreakerResistance=0.01  SnubberResistance=1e6  SnubberCapacitance=inf  Measurements=None  MoreParameters=on  NoBreakLoop=off
      settings: SourceProductName=Simscape Power Systems
  Step : Step  Time=start_time  SampleTime=0
  a : PMIOPort  Tag=PMCPort  Port=1  Side=Left
  b : PMIOPort  Tag=PMCPort  Port=2  Side=Left
  c : PMIOPort  Tag=PMCPort  Port=3  Side=Left
  A : PMIOPort  Tag=PMCPort  Port=4  Side=Right
  B : PMIOPort  Tag=PMCPort  Port=5  Side=Right
  C : PMIOPort  Tag=PMCPort  Port=6  Side=Right
  wires:
  Step/1 -> Breaker2/1, [step]
  [step] -> Breaker1/1
  [step] -> Breaker/1
  connections:
  A/RConn1 -- Breaker2/RConn1
  B/RConn1 -- Breaker/RConn1
  c/RConn1 -- Breaker1/LConn1
  C/RConn1 -- Breaker1/RConn1
  b/RConn1 -- Breaker/LConn1
  a/RConn1 -- Breaker2/LConn1

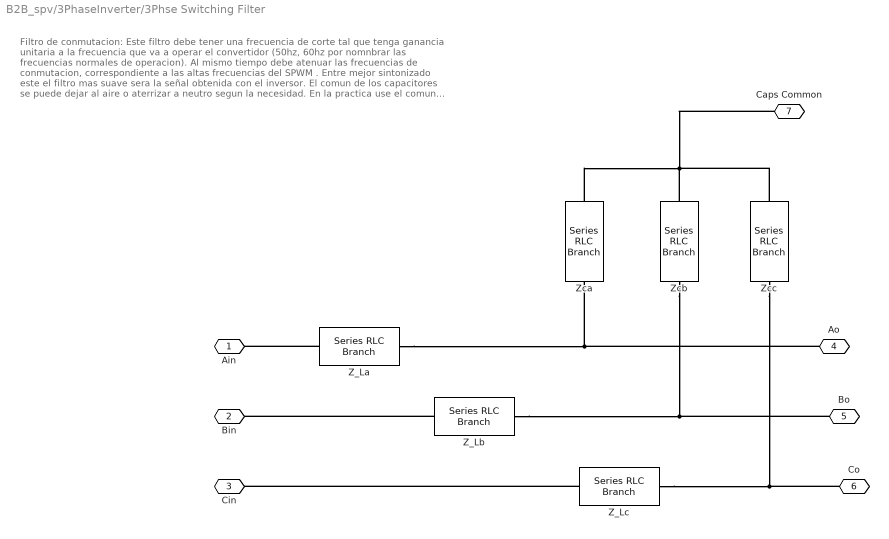
== system B2B_spv/3PhaseInverter/3Phse Switching Filter ==
  note: Filtro de conmutacion:
      | Este filtro debe tener una frecuencia de corte tal
      | que tenga ganancia unitaria a la frecuencia que va
      | a operar el convertidor (50hz, 60hz por nomnbrar
      | las frecuencias normales de operacion). Al mismo
      | tiempo debe atenuar las frecuencias de conmutacion,
      | correspondiente a las altas frecuencias del SPWM .
      | Entre mejor sintonizado este el filtro mas suave sera
      | la señal obtenida con el inversor. El comun de los
      | capacitores se puede dejar al aire o aterrizar a neutro
      | segun la necesidad. En la practica use el comun al
      | aire para un inversor trifasico de verdad y dio buenos
      | resultados.
  Z_La : powerlib/Elements/Series RLC Branch  LConnTagsString=__new0  RConnTagsString=__new0  BranchType=RL  Resistance=rLf  Inductance=Lf  SetiL0=off  InitialCurrent=0  Capacitance=2.2e-6  Setx0=off  InitialVoltage=0  Measurements=None
  Z_Lb : powerlib/Elements/Series RLC Branch  LConnTagsString=__new0  RConnTagsString=__new0  BranchType=RL  Resistance=rLf  Inductance=Lf  SetiL0=off  InitialCurrent=0  Capacitance=2.2e-6  Setx0=off  InitialVoltage=0  Measurements=None
  Z_Lc : powerlib/Elements/Series RLC Branch  LConnTagsString=__new0  RConnTagsString=__new0  BranchType=RL  Resistance=rLf  Inductance=Lf  SetiL0=off  InitialCurrent=0  Capacitance=2.2e-6  Setx0=off  InitialVoltage=0  Measurements=None
  Zca : powerlib/Elements/Series RLC Branch  LConnTagsString=__new0  RConnTagsString=__new0  BranchType=RC  Resistance=rCf  Inductance=1e-9  SetiL0=off  InitialCurrent=0  Capacitance=Cf  Setx0=off  InitialVoltage=0  Measurements=None
  Zcb : powerlib/Elements/Series RLC Branch  LConnTagsString=__new0  RConnTagsString=__new0  BranchType=RC  Resistance=rCf  Inductance=1e-9  SetiL0=off  InitialCurrent=0  Capacitance=Cf  Setx0=off  InitialVoltage=0  Measurements=None
  Zcc : powerlib/Elements/Series RLC Branch  LConnTagsString=__new0  RConnTagsString=__new0  BranchType=RC  Resistance=rCf  Inductance=1e-9  SetiL0=off  InitialCurrent=0  Capacitance=Cf  Setx0=off  InitialVoltage=0  Measurements=None
  Ain : PMIOPort  Port=1  Side=Left
  Bin : PMIOPort  Port=2  Side=Left
  Cin : PMIOPort  Port=3  Side=Left
  Ao : PMIOPort  Port=4  Side=Right
  Bo : PMIOPort  Port=5  Side=Right
  Co : PMIOPort  Port=6  Side=Right
  Caps Common : PMIOPort  Port=7  Side=Right
  connections:
  Zca/RConn1 -- Caps Common/RConn1 -- Zcc/RConn1 -- Zcb/RConn1
  Bo/RConn1 -- Zcb/LConn1 -- Z_Lb/RConn1
  Co/RConn1 -- Zcc/LConn1 -- Z_Lc/RConn1
  Ao/RConn1 -- Z_La/RConn1 -- Zca/LConn1
  Z_La/LConn1 -- Ain/RConn1
  Z_Lb/LConn1 -- Bin/RConn1
  Z_Lc/LConn1 -- Cin/RConn1

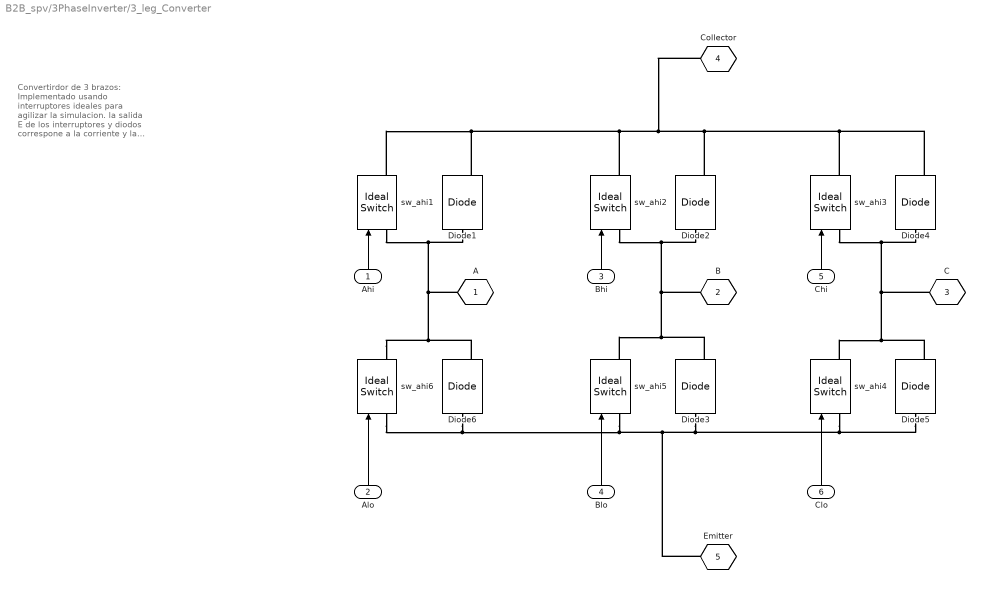
== system B2B_spv/3PhaseInverter/3_leg_Converter ==
  note: Convertirdor de 3 brazos:
      |
      | Implementado usando interruptores
      | ideales para agilizar la simulacion.
      | la salida E de los interruptores y diodos correspone
      | a la corriente y la tension de cada componente.
      |
      | si g=0 interruptor no conduce.
      | si g=1 interruptor conduce.
      |
      | conmutacion ocurre instantaneamente sin
      | retardo deacuerdo a la documentacion de matlab
  Ahi : Inport
  Alo : Inport  Port=2
  Bhi : Inport  Port=3
  Blo : Inport  Port=4
  Chi : Inport  Port=5
  Clo : Inport  Port=6
   sw_ahi{1..6} (6 alike) : powerlib/Power Electronics/Ideal Switch  Ron=20e-3  Lon=0  IC=0  Rs=1e6  Cs=10e-12  Measurements=on
  Diode{1..6} (6 alike) : powerlib/Power Electronics/Diode  Ron=.2  Lon=0  Vf=0.8  IC=0  UseSnubber=0  Rs=0  Cs=0  Measurements=on
  " A" : PMIOPort  Tag=PMCPort  Port=1  Side=Right
  B : PMIOPort  Tag=PMCPort  Port=2  Side=Right
  C : PMIOPort  Tag=PMCPort  Port=3  Side=Right
  Collector : PMIOPort  Tag=PMCPort  Port=4  Side=Right
  Emitter : PMIOPort  Tag=PMCPort  Port=5  Side=Right
  wires:
  Clo/1 -> " sw_ahi4"/1
  Alo/1 -> " sw_ahi6"/1
  Ahi/1 -> " sw_ahi1"/1
  Blo/1 -> " sw_ahi5"/1
  Bhi/1 -> " sw_ahi2"/1
  Chi/1 -> " sw_ahi3"/1
  connections:
  Diode3/RConn1 -- " sw_ahi5"/RConn1 -- B/RConn1 -- " sw_ahi2"/LConn1 -- Diode2/LConn1
  Diode3/LConn1 -- " sw_ahi4"/LConn1 -- Diode5/LConn1 -- Emitter/RConn1 -- " sw_ahi5"/LConn1 -- Diode6/LConn1 -- " sw_ahi6"/LConn1
  Diode2/RConn1 -- " sw_ahi3"/RConn1 -- Diode4/RConn1 -- Collector/RConn1 -- " sw_ahi2"/RConn1 -- " sw_ahi1"/RConn1 -- Diode1/RConn1
  " sw_ahi6"/RConn1 -- Diode6/RConn1 -- " A"/RConn1 -- " sw_ahi1"/LConn1 -- Diode1/LConn1
  " sw_ahi4"/RConn1 -- Diode5/RConn1 -- C/RConn1 -- " sw_ahi3"/LConn1 -- Diode4/LConn1

== system B2B_spv/3PhaseInverter/Steper1 ==
  In1 : Inport
  Product : Product
  Step : Step  Time=start_Delay  SampleTime=0
  Out1 : Outport
  wires:
  Step/1 -> Product/2
  In1/1 -> Product/1
  Product/1 -> Out1/1

== system B2B_spv/3PhaseInverter/Steper2 ==
  In1 : Inport
  Product : Product
  Step : Step  Time=start_Delay  SampleTime=0
  Out1 : Outport
  wires:
  Product/1 -> Out1/1
  In1/1 -> Product/1
  Step/1 -> Product/2

== system B2B_spv/3PhaseInverter/Steper3 ==
  In1 : Inport
  Product : Product
  Step : Step  Time=start_Delay  SampleTime=0
  Out1 : Outport
  wires:
  Product/1 -> Out1/1
  In1/1 -> Product/1
  Step/1 -> Product/2

== system B2B_spv/3PhaseInverter/Steper4 ==
  In1 : Inport
  Product : Product
  Step : Step  Time=start_Delay  SampleTime=0
  Out1 : Outport
  wires:
  Step/1 -> Product/2
  In1/1 -> Product/1
  Product/1 -> Out1/1

== system B2B_spv/3PhaseInverter/Steper5 ==
  In1 : Inport
  Product : Product
  Step : Step  Time=start_Delay  SampleTime=0
  Out1 : Outport
  wires:
  Product/1 -> Out1/1
  In1/1 -> Product/1
  Step/1 -> Product/2

== system B2B_spv/3PhaseInverter/Steper6 ==
  In1 : Inport
  Product : Product
  Step : Step  Time=start_Delay  SampleTime=0
  Out1 : Outport
  wires:
  Step/1 -> Product/2
  In1/1 -> Product/1
  Product/1 -> Out1/1

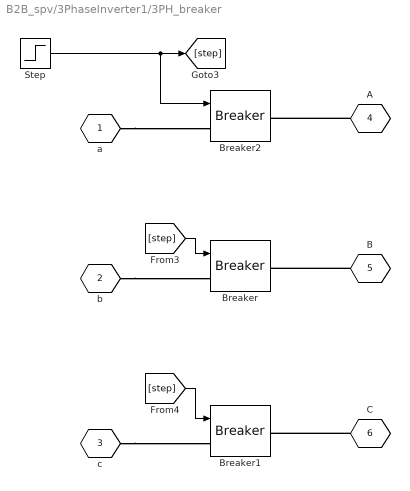
== system B2B_spv/3PhaseInverter1/3PH_breaker ==
  Breaker : powerlib/Elements/Breaker  InitialState=0  SwitchingTimes="[1/60  5/60]"  External=on  BreakerResistance=0.01  SnubberResistance=1e6  SnubberCapacitance=inf  Measurements=None  MoreParameters=on  NoBreakLoop=off
      settings: SourceProductName=Simscape Power Systems
  Breaker1 : powerlib/Elements/Breaker  InitialState=0  SwitchingTimes="[1/60  5/60]"  External=on  BreakerResistance=0.01  SnubberResistance=1e6  SnubberCapacitance=inf  Measurements=None  MoreParameters=on  NoBreakLoop=off
      settings: SourceProductName=Simscape Power Systems
  Breaker2 : powerlib/Elements/Breaker  InitialState=0  SwitchingTimes="[1/60  5/60]"  External=on  BreakerResistance=0.01  SnubberResistance=1e6  SnubberCapacitance=inf  Measurements=None  MoreParameters=on  NoBreakLoop=off
      settings: SourceProductName=Simscape Power Systems
  Step : Step  Time=start_time  SampleTime=0
  a : PMIOPort  Tag=PMCPort  Port=1  Side=Left
  b : PMIOPort  Tag=PMCPort  Port=2  Side=Left
  c : PMIOPort  Tag=PMCPort  Port=3  Side=Left
  A : PMIOPort  Tag=PMCPort  Port=4  Side=Right
  B : PMIOPort  Tag=PMCPort  Port=5  Side=Right
  C : PMIOPort  Tag=PMCPort  Port=6  Side=Right
  wires:
  [step] -> Breaker/1
  [step] -> Breaker1/1
  Step/1 -> [step], Breaker2/1
  connections:
  a/RConn1 -- Breaker2/LConn1
  b/RConn1 -- Breaker/LConn1
  C/RConn1 -- Breaker1/RConn1
  c/RConn1 -- Breaker1/LConn1
  B/RConn1 -- Breaker/RConn1
  A/RConn1 -- Breaker2/RConn1
